simulink model "FusionMODEL_version1"  (R2018a)
settings: Solver=FixedStepAuto  StartTime=0.0  StopTime=SimulationTime  FixedStep=SamplingTime  RelTol=1e-3
undefined symbols (not defined in the file or in its folder): ACTIVATE_CAM, ACTIVATE_RAD, CAM1_detTimeStamp, CAM1_MeasNoise, CAM1_objClassID, CAM1_PX, CAM1_PY, CAM1_VX, CAM1_VY, CAM2_detTimeStamp, CAM2_MeasNoise, CAM2_objClassID, CAM2_PX, CAM2_PY, CAM2_VX, CAM2_VY, CAM3_detTimeStamp, CAM3_MeasNoise, CAM3_objClassID, CAM3_PX, CAM3_PY, CAM3_VX, CAM3_VY, CAM4_detTimeStamp, CAM4_MeasNoise, CAM4_objClassID, CAM4_PX, CAM4_PY, CAM4_VX, CAM4_VY, CAM5_detTimeStamp, CAM5_MeasNoise, CAM5_objClassID, CAM5_PX, CAM5_PY, CAM5_VX, CAM5_VY, CAM6_detTimeStamp, CAM6_MeasNoise, CAM6_objClassID, CAM6_PX, CAM6_PY, CAM6_VX, CAM6_VY, CAM7_detTimeStamp, CAM7_MeasNoise, CAM7_objClassID, CAM7_PX, CAM7_PY, CAM7_VX, CAM7_VY, CAM8_detTimeStamp, CAM8_MeasNoise, CAM8_objClassID, CAM8_PX, CAM8_PY, CAM8_VX, CAM8_VY, CAM_nMeas, CAM_TYPE ... (+151)
libraries: simulink_extras x2
(part 6 of 6)

== system FusionMODEL_version1/SENSOR_MEASUREMENTS/RADAR_CAMERA_EGO_SENSOR_INTERFACE/RoadSensors/Camera6/ExtractMeasParam1 ==
  idx : Inport
  time : Inport  Port=2
  Constant : Constant  Value=LINE_CURVATURE_CAM6
  Constant1 : Constant  Value=LINE_CURVDERIVATIVE_CAM6
  Constant2 : Constant  Value=LINE_CURVELENGTH_CAM6
  Constant3 : Constant  Value=LINE_HEADINGANGLE_CAM6
  Constant4 : Constant  Value=LINE_LATERALOFFSET_CAM6
  Constant5 : Constant  Value=LINE_XMIN_CAM6
  Constant6 : Constant  Value=LINE_detTimeStamp_CAM6
  Constant7 : Constant  Value=LINE_XMAX_CAM6
  Constant8 : Constant  Value=LINE_WIDTH_CAM6
  CurvLength : Selector  NumberOfDimensions=2  InputPortWidth=3  IndexOptions=Index vector (port),Index vector (port)  Indices=[1 3],1  OutputSizes=1,1
  Curvature : Selector  NumberOfDimensions=2  InputPortWidth=3  IndexOptions=Index vector (port),Index vector (port)  Indices=[1 3],1  OutputSizes=1,1
  CurvatureRate : Selector  NumberOfDimensions=2  InputPortWidth=3  IndexOptions=Index vector (port),Index vector (port)  Indices=[1 3],1  OutputSizes=1,1
  HeadingAngle : Selector  NumberOfDimensions=2  InputPortWidth=3  IndexOptions=Index vector (port),Index vector (port)  Indices=[1 3],1  OutputSizes=1,1
  LateralOffset : Selector  NumberOfDimensions=2  InputPortWidth=3  IndexOptions=Index vector (port),Index vector (port)  Indices=[1 3],1  OutputSizes=1,1
  lineWidth : Selector  NumberOfDimensions=2  InputPortWidth=3  IndexOptions=Index vector (port),Index vector (port)  Indices=[1 3],1  OutputSizes=1,1
  minValidX : Selector  NumberOfDimensions=2  InputPortWidth=3  IndexOptions=Index vector (port),Index vector (port)  Indices=[1 3],1  OutputSizes=1,1
  minValidY : Selector  NumberOfDimensions=2  InputPortWidth=3  IndexOptions=Index vector (port),Index vector (port)  Indices=[1 3],1  OutputSizes=1,1
  timeStamp : Selector  NumberOfDimensions=2  InputPortWidth=3  IndexOptions=Select all,Index vector (port)  Indices=[1 3],1  OutputSizes=1,1
  curvature : Outport
  curvRate : Outport  Port=2
  curvLength : Outport  Port=3
  headingAngle : Outport  Port=4
  lateralOffset : Outport  Port=5
  xmin : Outport  Port=6
  xmax : Outport  Port=7
  lineMarkWidth : Outport  Port=8
  measCaptureTime : Outport  Port=9
  wires:
  Constant3/1 -> HeadingAngle/1
  Constant2/1 -> CurvLength/1
  HeadingAngle/1 -> headingAngle/1
  Constant/1 -> Curvature/1
  Constant1/1 -> CurvatureRate/1
  CurvLength/1 -> curvLength/1
  Curvature/1 -> curvature/1
  CurvatureRate/1 -> curvRate/1
  Constant4/1 -> LateralOffset/1
  Constant5/1 -> minValidX/1
  Constant6/1 -> timeStamp/1
  timeStamp/1 -> measCaptureTime/1
  minValidX/1 -> xmin/1
  LateralOffset/1 -> lateralOffset/1
  minValidY/1 -> xmax/1
  Constant7/1 -> minValidY/1
  lineWidth/1 -> lineMarkWidth/1
  time/1 -> minValidX/2, minValidY/2, lineWidth/2, timeStamp/2, LateralOffset/2, HeadingAngle/2, CurvLength/2, CurvatureRate/2, Curvature/2
  idx/1 -> minValidX/3, lineWidth/3, minValidY/3, LateralOffset/3, HeadingAngle/3, CurvLength/3, CurvatureRate/3, Curvature/3
  Constant8/1 -> lineWidth/1

== system FusionMODEL_version1/SENSOR_MEASUREMENTS/RADAR_CAMERA_EGO_SENSOR_INTERFACE/RoadSensors/Camera6/IsValid2 ==
  LineID : Inport
  curvature : Inport  Port=2
  curvatureRate : Inport  Port=3
  curvLength : Inport  Port=4
  HeadingAngle : Inport  Port=5
  Abs{,1..3} (4 alike) : Abs
  Add : Sum  Inputs=++++
  Constant : Constant  Value=uint16(0)
  Data Type Conversion : DataTypeConversion  OutDataTypeStr=uint16
  Switch : Switch  Threshold=0.000001
  validID : Outport
  wires:
  Add/1 -> Switch/2
  Abs2/1 -> Add/3
  Constant/1 -> Switch/3
  Abs/1 -> Add/1
  curvature/1 -> Abs/1
  Abs3/1 -> Add/4
  Abs1/1 -> Add/2
  HeadingAngle/1 -> Abs3/1
  curvatureRate/1 -> Abs1/1
  curvLength/1 -> Abs2/1
  LineID/1 -> Data Type Conversion/1
  Switch/1 -> validID/1
  Data Type Conversion/1 -> Switch/1

== system FusionMODEL_version1/SENSOR_MEASUREMENTS/RADAR_CAMERA_EGO_SENSOR_INTERFACE/RoadSensors/Camera6/Subsystem1 ==
  CameraLineCoeff : Inport
  curv : Inport  Port=2
  curvRate : Inport  Port=3
  curvLen : Inport  Port=4
  alpha : Inport  Port=5
  ValidID : Inport  Port=6
  lateralOffset : Inport  Port=7
  xmin : Inport  Port=8
  xmax : Inport  Port=9
  lineWidth : Inport  Port=10
  TIME_STAMP : Inport  Port=11
  iter : Inport  Port=12
  Assignment : Assignment  DiagnosticForDimensions=Warning  IndexOptions=Index vector (port)  Indices=1  OutputSizes=1
  Bus Creator1 : BusCreator  Inputs=11  OutDataTypeStr=Bus: LineMeasParam  NonVirtualBus=on
  Bus Creator2 : BusCreator  Inputs=11  OutDataTypeStr=Bus: LineMeasParam  NonVirtualBus=on
  Constant1 : Constant  Value=single(10)
  Constant14 : Constant  Value=uint8(6)
  Constant2 : Constant  Value=single(10)
  Constant{35..39,43} (6 alike) : Constant  Value=single(0)
  Constant44 : Constant  Value=single(10)
  Switch : Switch  Criteria=u2 ~= 0
  C1 : Outport
  wires:
  Bus Creator1/1 -> Switch/3
  ValidID/1 -> Bus Creator1/2, Switch/2, Bus Creator2/2  "lineID"
  Bus Creator2/1 -> Switch/1
  CameraLineCoeff/1 -> Assignment/1
  Switch/1 -> Assignment/2
  iter/1 -> Assignment/3
  Assignment/1 -> C1/1
  TIME_STAMP/1 -> Bus Creator2/1  "TimeStamp"
  curv/1 -> Bus Creator2/4  "curvature"
  curvRate/1 -> Bus Creator2/5  "curvatureRate"
  curvLen/1 -> Bus Creator2/6  "curveLength"
  alpha/1 -> Bus Creator2/7  "HeadingAngle"
  lateralOffset/1 -> Bus Creator2/8  "LateralOffset"
  lineWidth/1 -> Bus Creator2/11  "LineMarkWidth"
  xmax/1 -> Bus Creator2/10  "validMinLongCoordLine"
  xmin/1 -> Bus Creator2/9  "validMaxLongCoordLine"
  Constant35/1 -> Bus Creator1/1  "TimeStamp"
  Constant14/1 -> Bus Creator2/3, Bus Creator1/3  "cameraID"
  Constant36/1 -> Bus Creator1/4  "curvature"
  Constant37/1 -> Bus Creator1/5  "curvatureRate"
  Constant38/1 -> Bus Creator1/6  "curveLength"
  Constant39/1 -> Bus Creator1/7  "HeadingAngle"
  Constant43/1 -> Bus Creator1/8  "LateralOffset"
  Constant44/1 -> Bus Creator1/9  "validMaxLongCoordLine"
  Constant1/1 -> Bus Creator1/10  "validMinLongCoordLine"
  Constant2/1 -> Bus Creator1/11  "LineMarkWidth"

== system FusionMODEL_version1/SENSOR_MEASUREMENTS/RADAR_CAMERA_EGO_SENSOR_INTERFACE/RoadSensors/Camera7/ExtractMeasParam1 ==
  idx : Inport
  time : Inport  Port=2
  Constant : Constant  Value=LINE_CURVATURE_CAM7
  Constant1 : Constant  Value=LINE_CURVDERIVATIVE_CAM7
  Constant2 : Constant  Value=LINE_CURVELENGTH_CAM7
  Constant3 : Constant  Value=LINE_HEADINGANGLE_CAM7
  Constant4 : Constant  Value=LINE_LATERALOFFSET_CAM7
  Constant5 : Constant  Value=LINE_XMIN_CAM7
  Constant6 : Constant  Value=LINE_detTimeStamp_CAM7
  Constant7 : Constant  Value=LINE_XMAX_CAM7
  Constant8 : Constant  Value=LINE_WIDTH_CAM7
  CurvLength : Selector  NumberOfDimensions=2  InputPortWidth=3  IndexOptions=Index vector (port),Index vector (port)  Indices=[1 3],1  OutputSizes=1,1
  Curvature : Selector  NumberOfDimensions=2  InputPortWidth=3  IndexOptions=Index vector (port),Index vector (port)  Indices=[1 3],1  OutputSizes=1,1
  CurvatureRate : Selector  NumberOfDimensions=2  InputPortWidth=3  IndexOptions=Index vector (port),Index vector (port)  Indices=[1 3],1  OutputSizes=1,1
  HeadingAngle : Selector  NumberOfDimensions=2  InputPortWidth=3  IndexOptions=Index vector (port),Index vector (port)  Indices=[1 3],1  OutputSizes=1,1
  LateralOffset : Selector  NumberOfDimensions=2  InputPortWidth=3  IndexOptions=Index vector (port),Index vector (port)  Indices=[1 3],1  OutputSizes=1,1
  lineWidth : Selector  NumberOfDimensions=2  InputPortWidth=3  IndexOptions=Index vector (port),Index vector (port)  Indices=[1 3],1  OutputSizes=1,1
  minValidX : Selector  NumberOfDimensions=2  InputPortWidth=3  IndexOptions=Index vector (port),Index vector (port)  Indices=[1 3],1  OutputSizes=1,1
  minValidY : Selector  NumberOfDimensions=2  InputPortWidth=3  IndexOptions=Index vector (port),Index vector (port)  Indices=[1 3],1  OutputSizes=1,1
  timeStamp : Selector  NumberOfDimensions=2  InputPortWidth=3  IndexOptions=Select all,Index vector (port)  Indices=[1 3],1  OutputSizes=1,1
  curvature : Outport
  curvRate : Outport  Port=2
  curvLength : Outport  Port=3
  headingAngle : Outport  Port=4
  lateralOffset : Outport  Port=5
  xmin : Outport  Port=6
  xmax : Outport  Port=7
  lineMarkWidth : Outport  Port=8
  measCaptureTime : Outport  Port=9
  wires:
  Constant3/1 -> HeadingAngle/1
  Constant2/1 -> CurvLength/1
  HeadingAngle/1 -> headingAngle/1
  Constant/1 -> Curvature/1
  Constant1/1 -> CurvatureRate/1
  CurvLength/1 -> curvLength/1
  Curvature/1 -> curvature/1
  CurvatureRate/1 -> curvRate/1
  Constant4/1 -> LateralOffset/1
  Constant5/1 -> minValidX/1
  Constant6/1 -> timeStamp/1
  timeStamp/1 -> measCaptureTime/1
  minValidX/1 -> xmin/1
  LateralOffset/1 -> lateralOffset/1
  minValidY/1 -> xmax/1
  Constant7/1 -> minValidY/1
  lineWidth/1 -> lineMarkWidth/1
  time/1 -> minValidX/2, minValidY/2, lineWidth/2, timeStamp/2, LateralOffset/2, HeadingAngle/2, CurvLength/2, CurvatureRate/2, Curvature/2
  idx/1 -> minValidX/3, lineWidth/3, minValidY/3, LateralOffset/3, HeadingAngle/3, CurvLength/3, CurvatureRate/3, Curvature/3
  Constant8/1 -> lineWidth/1

== system FusionMODEL_version1/SENSOR_MEASUREMENTS/RADAR_CAMERA_EGO_SENSOR_INTERFACE/RoadSensors/Camera7/IsValid2 ==
  LineID : Inport
  curvature : Inport  Port=2
  curvatureRate : Inport  Port=3
  curvLength : Inport  Port=4
  HeadingAngle : Inport  Port=5
  Abs{,1..3} (4 alike) : Abs
  Add : Sum  Inputs=++++
  Constant : Constant  Value=uint16(0)
  Data Type Conversion : DataTypeConversion  OutDataTypeStr=uint16
  Switch : Switch  Threshold=0.000001
  validID : Outport
  wires:
  Add/1 -> Switch/2
  Abs2/1 -> Add/3
  Constant/1 -> Switch/3
  Abs/1 -> Add/1
  curvature/1 -> Abs/1
  Abs3/1 -> Add/4
  Abs1/1 -> Add/2
  HeadingAngle/1 -> Abs3/1
  curvatureRate/1 -> Abs1/1
  curvLength/1 -> Abs2/1
  LineID/1 -> Data Type Conversion/1
  Switch/1 -> validID/1
  Data Type Conversion/1 -> Switch/1

== system FusionMODEL_version1/SENSOR_MEASUREMENTS/RADAR_CAMERA_EGO_SENSOR_INTERFACE/RoadSensors/Camera7/Subsystem1 ==
  CameraLineCoeff : Inport
  curv : Inport  Port=2
  curvRate : Inport  Port=3
  curvLen : Inport  Port=4
  alpha : Inport  Port=5
  ValidID : Inport  Port=6
  lateralOffset : Inport  Port=7
  xmin : Inport  Port=8
  xmax : Inport  Port=9
  lineWidth : Inport  Port=10
  TIME_STAMP : Inport  Port=11
  iter : Inport  Port=12
  Assignment : Assignment  DiagnosticForDimensions=Warning  IndexOptions=Index vector (port)  Indices=1  OutputSizes=1
  Bus Creator1 : BusCreator  Inputs=11  OutDataTypeStr=Bus: LineMeasParam  NonVirtualBus=on
  Bus Creator2 : BusCreator  Inputs=11  OutDataTypeStr=Bus: LineMeasParam  NonVirtualBus=on
  Constant1 : Constant  Value=single(10)
  Constant14 : Constant  Value=uint8(7)
  Constant2 : Constant  Value=single(10)
  Constant{35..39,43} (6 alike) : Constant  Value=single(0)
  Constant44 : Constant  Value=single(10)
  Switch : Switch  Criteria=u2 ~= 0
  C1 : Outport
  wires:
  Bus Creator1/1 -> Switch/3
  ValidID/1 -> Bus Creator1/2, Switch/2, Bus Creator2/2  "lineID"
  Bus Creator2/1 -> Switch/1
  CameraLineCoeff/1 -> Assignment/1
  Switch/1 -> Assignment/2
  iter/1 -> Assignment/3
  Assignment/1 -> C1/1
  TIME_STAMP/1 -> Bus Creator2/1  "TimeStamp"
  curv/1 -> Bus Creator2/4  "curvature"
  curvRate/1 -> Bus Creator2/5  "curvatureRate"
  curvLen/1 -> Bus Creator2/6  "curveLength"
  alpha/1 -> Bus Creator2/7  "HeadingAngle"
  lateralOffset/1 -> Bus Creator2/8  "LateralOffset"
  lineWidth/1 -> Bus Creator2/11  "LineMarkWidth"
  xmax/1 -> Bus Creator2/10  "validMinLongCoordLine"
  xmin/1 -> Bus Creator2/9  "validMaxLongCoordLine"
  Constant35/1 -> Bus Creator1/1  "TimeStamp"
  Constant14/1 -> Bus Creator2/3, Bus Creator1/3  "cameraID"
  Constant36/1 -> Bus Creator1/4  "curvature"
  Constant37/1 -> Bus Creator1/5  "curvatureRate"
  Constant38/1 -> Bus Creator1/6  "curveLength"
  Constant39/1 -> Bus Creator1/7  "HeadingAngle"
  Constant43/1 -> Bus Creator1/8  "LateralOffset"
  Constant44/1 -> Bus Creator1/9  "validMaxLongCoordLine"
  Constant1/1 -> Bus Creator1/10  "validMinLongCoordLine"
  Constant2/1 -> Bus Creator1/11  "LineMarkWidth"

== system FusionMODEL_version1/SENSOR_MEASUREMENTS/RADAR_CAMERA_EGO_SENSOR_INTERFACE/RoadSensors/Camera8/ExtractMeasParam1 ==
  idx : Inport
  time : Inport  Port=2
  Constant : Constant  Value=LINE_CURVATURE_CAM8
  Constant1 : Constant  Value=LINE_CURVDERIVATIVE_CAM8
  Constant2 : Constant  Value=LINE_CURVELENGTH_CAM8
  Constant3 : Constant  Value=LINE_HEADINGANGLE_CAM8
  Constant4 : Constant  Value=LINE_LATERALOFFSET_CAM8
  Constant5 : Constant  Value=LINE_XMIN_CAM8
  Constant6 : Constant  Value=LINE_detTimeStamp_CAM8
  Constant7 : Constant  Value=LINE_XMAX_CAM8
  Constant8 : Constant  Value=LINE_WIDTH_CAM8
  CurvLength : Selector  NumberOfDimensions=2  InputPortWidth=3  IndexOptions=Index vector (port),Index vector (port)  Indices=[1 3],1  OutputSizes=1,1
  Curvature : Selector  NumberOfDimensions=2  InputPortWidth=3  IndexOptions=Index vector (port),Index vector (port)  Indices=[1 3],1  OutputSizes=1,1
  CurvatureRate : Selector  NumberOfDimensions=2  InputPortWidth=3  IndexOptions=Index vector (port),Index vector (port)  Indices=[1 3],1  OutputSizes=1,1
  HeadingAngle : Selector  NumberOfDimensions=2  InputPortWidth=3  IndexOptions=Index vector (port),Index vector (port)  Indices=[1 3],1  OutputSizes=1,1
  LateralOffset : Selector  NumberOfDimensions=2  InputPortWidth=3  IndexOptions=Index vector (port),Index vector (port)  Indices=[1 3],1  OutputSizes=1,1
  lineWidth : Selector  NumberOfDimensions=2  InputPortWidth=3  IndexOptions=Index vector (port),Index vector (port)  Indices=[1 3],1  OutputSizes=1,1
  minValidX : Selector  NumberOfDimensions=2  InputPortWidth=3  IndexOptions=Index vector (port),Index vector (port)  Indices=[1 3],1  OutputSizes=1,1
  minValidY : Selector  NumberOfDimensions=2  InputPortWidth=3  IndexOptions=Index vector (port),Index vector (port)  Indices=[1 3],1  OutputSizes=1,1
  timeStamp : Selector  NumberOfDimensions=2  InputPortWidth=3  IndexOptions=Select all,Index vector (port)  Indices=[1 3],1  OutputSizes=1,1
  curvature : Outport
  curvRate : Outport  Port=2
  curvLength : Outport  Port=3
  headingAngle : Outport  Port=4
  lateralOffset : Outport  Port=5
  xmin : Outport  Port=6
  xmax : Outport  Port=7
  lineMarkWidth : Outport  Port=8
  measCaptureTime : Outport  Port=9
  wires:
  Constant3/1 -> HeadingAngle/1
  Constant2/1 -> CurvLength/1
  HeadingAngle/1 -> headingAngle/1
  Constant/1 -> Curvature/1
  Constant1/1 -> CurvatureRate/1
  CurvLength/1 -> curvLength/1
  Curvature/1 -> curvature/1
  CurvatureRate/1 -> curvRate/1
  Constant4/1 -> LateralOffset/1
  Constant5/1 -> minValidX/1
  Constant6/1 -> timeStamp/1
  timeStamp/1 -> measCaptureTime/1
  minValidX/1 -> xmin/1
  LateralOffset/1 -> lateralOffset/1
  minValidY/1 -> xmax/1
  Constant7/1 -> minValidY/1
  lineWidth/1 -> lineMarkWidth/1
  time/1 -> minValidX/2, minValidY/2, lineWidth/2, timeStamp/2, LateralOffset/2, HeadingAngle/2, CurvLength/2, CurvatureRate/2, Curvature/2
  idx/1 -> minValidX/3, lineWidth/3, minValidY/3, LateralOffset/3, HeadingAngle/3, CurvLength/3, CurvatureRate/3, Curvature/3
  Constant8/1 -> lineWidth/1

== system FusionMODEL_version1/SENSOR_MEASUREMENTS/RADAR_CAMERA_EGO_SENSOR_INTERFACE/RoadSensors/Camera8/IsValid2 ==
  LineID : Inport
  curvature : Inport  Port=2
  curvatureRate : Inport  Port=3
  curvLength : Inport  Port=4
  HeadingAngle : Inport  Port=5
  Abs{,1..3} (4 alike) : Abs
  Add : Sum  Inputs=++++
  Constant : Constant  Value=uint16(0)
  Data Type Conversion : DataTypeConversion  OutDataTypeStr=uint16
  Switch : Switch  Threshold=0.000001
  validID : Outport
  wires:
  Add/1 -> Switch/2
  Abs2/1 -> Add/3
  Constant/1 -> Switch/3
  Abs/1 -> Add/1
  curvature/1 -> Abs/1
  Abs3/1 -> Add/4
  Abs1/1 -> Add/2
  HeadingAngle/1 -> Abs3/1
  curvatureRate/1 -> Abs1/1
  curvLength/1 -> Abs2/1
  LineID/1 -> Data Type Conversion/1
  Switch/1 -> validID/1
  Data Type Conversion/1 -> Switch/1

== system FusionMODEL_version1/SENSOR_MEASUREMENTS/RADAR_CAMERA_EGO_SENSOR_INTERFACE/RoadSensors/Camera8/Subsystem1 ==
  CameraLineCoeff : Inport
  curv : Inport  Port=2
  curvRate : Inport  Port=3
  curvLen : Inport  Port=4
  alpha : Inport  Port=5
  ValidID : Inport  Port=6
  lateralOffset : Inport  Port=7
  xmin : Inport  Port=8
  xmax : Inport  Port=9
  lineWidth : Inport  Port=10
  TIME_STAMP : Inport  Port=11
  iter : Inport  Port=12
  Assignment : Assignment  DiagnosticForDimensions=Warning  IndexOptions=Index vector (port)  Indices=1  OutputSizes=1
  Bus Creator1 : BusCreator  Inputs=11  OutDataTypeStr=Bus: LineMeasParam  NonVirtualBus=on
  Bus Creator2 : BusCreator  Inputs=11  OutDataTypeStr=Bus: LineMeasParam  NonVirtualBus=on
  Constant1 : Constant  Value=single(10)
  Constant14 : Constant  Value=uint8(8)
  Constant2 : Constant  Value=single(10)
  Constant{35..39,43} (6 alike) : Constant  Value=single(0)
  Constant44 : Constant  Value=single(10)
  Switch : Switch  Criteria=u2 ~= 0
  C1 : Outport
  wires:
  Bus Creator1/1 -> Switch/3
  ValidID/1 -> Bus Creator1/2, Switch/2, Bus Creator2/2  "lineID"
  Bus Creator2/1 -> Switch/1
  CameraLineCoeff/1 -> Assignment/1
  Switch/1 -> Assignment/2
  iter/1 -> Assignment/3
  Assignment/1 -> C1/1
  TIME_STAMP/1 -> Bus Creator2/1  "TimeStamp"
  curv/1 -> Bus Creator2/4  "curvature"
  curvRate/1 -> Bus Creator2/5  "curvatureRate"
  curvLen/1 -> Bus Creator2/6  "curveLength"
  alpha/1 -> Bus Creator2/7  "HeadingAngle"
  lateralOffset/1 -> Bus Creator2/8  "LateralOffset"
  lineWidth/1 -> Bus Creator2/11  "LineMarkWidth"
  xmax/1 -> Bus Creator2/10  "validMinLongCoordLine"
  xmin/1 -> Bus Creator2/9  "validMaxLongCoordLine"
  Constant35/1 -> Bus Creator1/1  "TimeStamp"
  Constant14/1 -> Bus Creator2/3, Bus Creator1/3  "cameraID"
  Constant36/1 -> Bus Creator1/4  "curvature"
  Constant37/1 -> Bus Creator1/5  "curvatureRate"
  Constant38/1 -> Bus Creator1/6  "curveLength"
  Constant39/1 -> Bus Creator1/7  "HeadingAngle"
  Constant43/1 -> Bus Creator1/8  "LateralOffset"
  Constant44/1 -> Bus Creator1/9  "validMaxLongCoordLine"
  Constant1/1 -> Bus Creator1/10  "validMinLongCoordLine"
  Constant2/1 -> Bus Creator1/11  "LineMarkWidth"

== system FusionMODEL_version1/OBJECT_TRACKER_SENSOR_FUSION/SET_SENSOR_CALLIBRATION_PARAMETER/SET_CAMERA_SENSOR_PARAM/SET_CAMERA_EXTRINSIC_PARAM/SET_CAMERA_EXTRINSIC_PARAM/CreateRotationMatTranslationVector ==
  yawInstall : Inport
  xMount : Inport  Port=2
  yMount : Inport  Port=3
  Cos : Trigonometry  Operator=cos
  Cos2 : Trigonometry
  Degrees to Radians : simulink_extras/Transformations/Degrees to Radians
  Gain1 : Gain  Gain=-1
  Gain2 : Gain  Gain=ROT_CONVENTION
  Mux : Mux
  Mux1 : Mux  Inputs=2
  Reshape : Reshape  OutputDimensionality=Customize  OutputDimensions=[2 2]
  Reshape1 : Reshape  OutputDimensionality=Column vector (2-D)  OutputDimensions=[2 2]
  RotMatrx : Outport
  TranslationVector : Outport  Port=2
  wires:
  Cos/1 -> [cos_theta], Mux/1
  [cos_theta] -> Mux/4
  Reshape/1 -> RotMatrx/1
  Degrees to Radians/1 -> Cos2/1, Cos/1
  Mux/1 -> Reshape/1
  Cos2/1 -> Mux/2, Gain1/1
  xMount/1 -> Mux1/1
  yMount/1 -> Mux1/2
  Mux1/1 -> Reshape1/1
  Reshape1/1 -> TranslationVector/1
  Gain1/1 -> Mux/3
  yawInstall/1 -> Gain2/1
  Gain2/1 -> Degrees to Radians/1

== system FusionMODEL_version1/OBJECT_TRACKER_SENSOR_FUSION/SET_SENSOR_CALLIBRATION_PARAMETER/SET_RADAR_SENSOR_PARAM/SET_RADAR_EXTRINSIC_PARAM/SET_RADAR_EXTRINSIC_PARAM/CREATE_ROTATION_MATRIX_TRANSLATION_VECTOR ==
  yawInstall : Inport
  xMount : Inport  Port=2
  yMount : Inport  Port=3
  Cos : Trigonometry  Operator=cos
  Cos2 : Trigonometry
  Degrees to Radians : simulink_extras/Transformations/Degrees to Radians
  Gain1 : Gain  Gain=-1
  Gain2 : Gain  Gain=ROT_CONVENTION
  Mux : Mux
  Mux1 : Mux  Inputs=2
  Reshape : Reshape  OutputDimensionality=Customize  OutputDimensions=[2 2]
  Reshape1 : Reshape  OutputDimensionality=Column vector (2-D)  OutputDimensions=[2 2]
  RotMatrx : Outport
  TranslationVector : Outport  Port=2
  wires:
  Cos/1 -> [cos_theta], Mux/1
  [cos_theta] -> Mux/4
  Reshape/1 -> RotMatrx/1
  Degrees to Radians/1 -> Cos2/1, Cos/1
  Mux/1 -> Reshape/1
  Cos2/1 -> Mux/2, Gain1/1
  xMount/1 -> Mux1/1
  yMount/1 -> Mux1/2
  Mux1/1 -> Reshape1/1
  Reshape1/1 -> TranslationVector/1
  Gain1/1 -> Mux/3
  yawInstall/1 -> Gain2/1
  Gain2/1 -> Degrees to Radians/1

== system FusionMODEL_version1/OBJECT_TRACKER_SENSOR_FUSION/SPATIAL_ALLIGNMENT/CAMERA_MEASUREMENTS_SPATIAL_ALLIGNMENT/For Iterator Subsystem/For Iterator Subsystem/CoordinateTransformation1 ==
  meas : Inport
  SensorParam : Inport  Port=2
  Action Port : ActionPort  ActionType=then
  InfoExtractor : Subsystem
  Meas_Noise_Cov_Transformation : Subsystem
  Position_Transformation : Subsystem
  Subsystem : Subsystem
  Velocity_Transformation : Subsystem
  measUpd : Outport
  wires:
  meas/1 -> InfoExtractor/1(In1)
  SensorParam/1 -> InfoExtractor/2(In2)
  Velocity_Transformation/1(VelXcts) -> [VxCTS]  "vxCTS"
  InfoExtractor/5(RotMat2D) -> Velocity_Transformation/3(RotMatrix2D), Meas_Noise_Cov_Transformation/1(RotMatrix), [RotMat]
  InfoExtractor/4(<vy>) -> Velocity_Transformation/2(Vy)
  InfoExtractor/3(<vx>) -> Velocity_Transformation/1(Vx)
  InfoExtractor/1(<px>) -> Position_Transformation/1(Px)
  InfoExtractor/2(<py>) -> Position_Transformation/2(Py)
  InfoExtractor/7(MeasNoiseCov) -> Meas_Noise_Cov_Transformation/2(MeasCovarience)
  [RotMat] -> Position_Transformation/3(RotationMat)
  [TransVector] -> Position_Transformation/4(TranslationVector)
  InfoExtractor/6(TransVec2D) -> [TransVector]
  Position_Transformation/1(PosXcts) -> Subsystem/1(pxCTS)
  Meas_Noise_Cov_Transformation/1(MeasCovTransformed) -> Subsystem/5(covCTS)
  Position_Transformation/2(PosYcts) -> Subsystem/2(pyCTS)
  Velocity_Transformation/2(VelYcts) -> [VyCTS]  "vyCTS"
  [VxCTS] -> Subsystem/3(vxCTS)
  [VyCTS] -> Subsystem/4(vyCTS)
  Subsystem/1(measUpd) -> measUpd/1

== system FusionMODEL_version1/OBJECT_TRACKER_SENSOR_FUSION/SPATIAL_ALLIGNMENT/CAMERA_MEASUREMENTS_SPATIAL_ALLIGNMENT/For Iterator Subsystem/For Iterator Subsystem/SetMeasurement ==
  measTransformed : Inport
  measID : Inport  Port=2
  CamCANidx : Inport  Port=3
  CameraMeasCAN : Inport  Port=4
  CameraMeasCTSMat : Inport  Port=5
  Assignment1 : Assignment  NumberOfDimensions=2  DiagnosticForDimensions=Warning  IndexOptions=Index vector (dialog),Index vector (port)  Indices=1:8,1  OutputSizes=1,1
  Bus Selector : BusSelector  OutputSignals=measID,cameraID
  Bus to Vector : BusToVector
  Constant : Constant  Value=single(zeros(8,1))
  Data Type Conversion : DataTypeConversion  OutDataTypeStr=single
  Data Type Conversion1 : DataTypeConversion  OutDataTypeStr=single
  Mux : Mux  Inputs=3
  Reshape : Reshape  OutputDimensionality=Column vector (2-D)
  Switch : Switch  Criteria=u2 ~= 0
  Unit Delay : UnitDelay  InitialCondition=single(zeros(8, 200))  SampleTime=-1
  CameraCTSMatUpd : Outport
  wires:
  CameraMeasCTSMat/1 -> Unit Delay/1
  measID/1 -> Switch/2
  Constant/1 -> Switch/3
  Switch/1 -> Assignment1/2
  CamCANidx/1 -> Assignment1/3
  CameraMeasCAN/1 -> Bus Selector/1
  Unit Delay/1 -> Assignment1/1
  measTransformed/1 -> Bus to Vector/1
  Assignment1/1 -> CameraCTSMatUpd/1
  Bus Selector/1 -> Data Type Conversion/1  "<measID>"
  Bus Selector/2 -> Data Type Conversion1/1  "<cameraID>"
  Data Type Conversion1/1 -> Mux/3
  Data Type Conversion/1 -> Mux/2
  Bus to Vector/1 -> Mux/1
  Mux/1 -> Reshape/1
  Reshape/1 -> Switch/1

== system FusionMODEL_version1/OBJECT_TRACKER_SENSOR_FUSION/SPATIAL_ALLIGNMENT/CAMERA_MEASUREMENTS_SPATIAL_ALLIGNMENT/For Iterator Subsystem/For Iterator Subsystem/SetMeasurement1 ==
  measTransformed : Inport
  measID : Inport  Port=2
  CamCANidx : Inport  Port=3
  CameraMeasCAN : Inport  Port=4
  CameraMeasCTSMat : Inport  Port=5
  CameraMeasCTSNoiseMat : Inport  Port=6
  CameraMeasCTSRef : Inport  Port=7
  Assignment1 : Assignment  NumberOfDimensions=2  DiagnosticForDimensions=Warning  IndexOptions=Assign all,Index vector (port)  Indices=1:2,1  OutputSizes=1,1
  Assignment2 : Assignment  NumberOfDimensions=3  DiagnosticForDimensions=Warning  IndexOptions=Assign all,Assign all,Index vector (port)  Indices=1:8,1,1  OutputSizes=1,1,1
  Assignment3 : Assignment  NumberOfDimensions=2  DiagnosticForDimensions=Warning  IndexOptions=Assign all,Index vector (port)  Indices=1:8,1  OutputSizes=1,1
  Bus Selector : BusSelector  OutputSignals=measID,cameraID
  Bus Selector1 : BusSelector  OutputSignals=stateCTS,covCTS
  Constant : Constant  Value=single(zeros(2,1))
  Constant1 : Constant  Value=single(zeros(2,2))
  Constant2 : Constant  Value=uint16(zeros(2,1))
  Data Type Conversion : DataTypeConversion  OutDataTypeStr=uint16
  Mux : Mux  Inputs=2
  Reshape : Reshape  OutputDimensionality=Column vector (2-D)
  Switch : Switch  Criteria=u2 ~= 0
  Switch1 : Switch  Criteria=u2 ~= 0
  Switch2 : Switch  Criteria=u2 ~= 0
  Unit Delay : UnitDelay  InitialCondition=single(zeros(2, 200))  SampleTime=-1
  Unit Delay1 : UnitDelay  InitialCondition=single(zeros(2, 2, 200))  SampleTime=-1
  Unit Delay2 : UnitDelay  InitialCondition=uint16(zeros(2, 200))  SampleTime=-1
  CameraCTSMatUpd : Outport
  CameraCTSNoiseCovMatUpd : Outport  Port=2
  CameraCTSRefUpd : Outport  Port=3
  wires:
  CameraMeasCTSMat/1 -> Unit Delay/1
  measID/1 -> Switch/2, Switch2/2, Switch1/2
  Constant/1 -> Switch/3
  Switch/1 -> Assignment1/2
  CamCANidx/1 -> [idx], Assignment1/3
  CameraMeasCAN/1 -> Bus Selector/1
  Unit Delay/1 -> Assignment1/1
  Assignment1/1 -> CameraCTSMatUpd/1
  Bus Selector/1 -> Mux/1  "<measID>"
  Bus Selector/2 -> Data Type Conversion/1  "<cameraID>"
  Mux/1 -> Reshape/1
  CameraMeasCTSNoiseMat/1 -> Unit Delay1/1
  Unit Delay1/1 -> Assignment2/1
  Switch1/1 -> Assignment2/2
  measTransformed/1 -> Bus Selector1/1
  Bus Selector1/1 -> Switch/1  "<stateCTS>"
  Constant1/1 -> Switch1/3
  Bus Selector1/2 -> [CTSNoiseCov]  "<covCTS>"
  [CTSNoiseCov] -> Switch1/1
  [idx] -> Assignment2/3
  Switch2/1 -> Assignment3/2
  Constant2/1 -> Switch2/3
  [idx] -> Assignment3/3
  Unit Delay2/1 -> Assignment3/1
  CameraMeasCTSRef/1 -> Unit Delay2/1
  Reshape/1 -> [CTSRef]
  [CTSRef] -> Switch2/1
  Assignment2/1 -> CameraCTSNoiseCovMatUpd/1
  Assignment3/1 -> CameraCTSRefUpd/1
  Data Type Conversion/1 -> Mux/2

== system FusionMODEL_version1/OBJECT_TRACKER_SENSOR_FUSION/SPATIAL_ALLIGNMENT/CAMERA_MEASUREMENTS_SPATIAL_ALLIGNMENT/For Iterator Subsystem/For Iterator Subsystem/Subsystem ==
  measCAN : Inport
  measIdx : Inport  Port=2
  Add : Sum
  Bus Selector : BusSelector  OutputSignals=measID
  Constant : Constant  Value=int32(0)
  Constant2 : Constant  Value=int32(1)
  If : If  IfExpression=u1 ~= 0  ShowElse=off
  Selector : Selector  NumberOfDimensions=2  InputPortWidth=3  IndexOptions=Select all,Index vector (port)  Indices=[1 3],1  OutputSizes=1,1
  Switch : Switch  Criteria=u2 ~= 0
  Unit Delay : UnitDelay  InitialCondition=int32(0)  SampleTime=-1
  isValid : Outport
  measID : Outport  Port=2
  nValidMeasCnt : Outport  Port=3
  meas_i : Outport  Port=4
  wires:
  measIdx/1 -> Selector/2
  Selector/1 -> meas_i/1, Bus Selector/1
  measCAN/1 -> Selector/1
  If/1 -> isValid/1
  Switch/1 -> Add/1
  Bus Selector/1 -> measID/1, If/1, Switch/2  "<measID>"
  Constant2/1 -> Switch/1
  Unit Delay/1 -> Add/2
  Constant/1 -> Switch/3
  Add/1 -> nValidMeasCnt/1, Unit Delay/1

== system FusionMODEL_version1/OBJECT_TRACKER_SENSOR_FUSION/SPATIAL_ALLIGNMENT/RADAR_MEASUREMENTS_SPATIAL_ALLIGNMENT/RADAR_MEASUREMENTS_SPATIAL_ALLIGNMENT/COORDINATE_TRANSFORMATION/COORDINATE_TRANSFORMATION ==
  meas : Inport
  SensorParam : Inport  Port=2
  Action Port : ActionPort  ActionType=then
  GET_DATA : Subsystem
  MEAS_NOISE_COV_TRANSFORMATION : Subsystem
  POSITION_TRANSFORMATION : Subsystem
  SET_DATA : Subsystem
  VELOCITY_TRANSFORMATION : Subsystem
  measUpd : Outport
  wires:
  meas/1 -> GET_DATA/1(In1)
  SensorParam/1 -> GET_DATA/2(In2)
  VELOCITY_TRANSFORMATION/1(VelXcts) -> [VxCTS]  "vxCTS"
  GET_DATA/5(RotMat2D) -> VELOCITY_TRANSFORMATION/3(RotMatrix2D), MEAS_NOISE_COV_TRANSFORMATION/1(RotMatrix), [RotMat]
  GET_DATA/4(<vy>) -> VELOCITY_TRANSFORMATION/2(Vy)
  GET_DATA/3(<vx>) -> VELOCITY_TRANSFORMATION/1(Vx)
  GET_DATA/1(<px>) -> POSITION_TRANSFORMATION/1(Px)
  GET_DATA/2(<py>) -> POSITION_TRANSFORMATION/2(Py)
  GET_DATA/7(MeasNoiseCov) -> MEAS_NOISE_COV_TRANSFORMATION/2(MeasCovarience)
  [RotMat] -> POSITION_TRANSFORMATION/3(RotationMat)
  [TransVector] -> POSITION_TRANSFORMATION/4(TranslationVector)
  GET_DATA/6(TransVec2D) -> [TransVector]
  POSITION_TRANSFORMATION/1(PosXcts) -> SET_DATA/1(pxCTS)
  MEAS_NOISE_COV_TRANSFORMATION/1(MeasCovTransformed) -> SET_DATA/5(covCTS)
  POSITION_TRANSFORMATION/2(PosYcts) -> SET_DATA/2(pyCTS)
  VELOCITY_TRANSFORMATION/2(VelYcts) -> [VyCTS]  "vyCTS"
  [VxCTS] -> SET_DATA/3(vxCTS)
  [VyCTS] -> SET_DATA/4(vyCTS)
  SET_DATA/1(measUpd) -> measUpd/1

== system FusionMODEL_version1/OBJECT_TRACKER_SENSOR_FUSION/SPATIAL_ALLIGNMENT/RADAR_MEASUREMENTS_SPATIAL_ALLIGNMENT/RADAR_MEASUREMENTS_SPATIAL_ALLIGNMENT/COORDINATE_TRANSFORMATION/GET_DATA ==
  measCAN : Inport
  measIdx : Inport  Port=2
  Add : Sum
  Bus Selector : BusSelector  OutputSignals=measID
  Constant : Constant  Value=int32(0)
  Constant2 : Constant  Value=int32(1)
  If : If  IfExpression=u1 ~= 0  ShowElse=off
  Selector : Selector  NumberOfDimensions=2  InputPortWidth=3  IndexOptions=Select all,Index vector (port)  Indices=[1 3],1  OutputSizes=1,1
  Switch : Switch  Criteria=u2 ~= 0
  Unit Delay : UnitDelay  InitialCondition=int32(0)  SampleTime=-1
  isValid : Outport
  measID : Outport  Port=2
  nValidMeasCnt : Outport  Port=3
  meas_i : Outport  Port=4
  wires:
  measIdx/1 -> Selector/2
  Selector/1 -> meas_i/1, Bus Selector/1
  measCAN/1 -> Selector/1
  If/1 -> isValid/1
  Switch/1 -> Add/1
  Bus Selector/1 -> measID/1, If/1, Switch/2  "<measID>"
  Constant2/1 -> Switch/1
  Unit Delay/1 -> Add/2
  Constant/1 -> Switch/3
  Add/1 -> nValidMeasCnt/1, Unit Delay/1

== system FusionMODEL_version1/OBJECT_TRACKER_SENSOR_FUSION/SPATIAL_ALLIGNMENT/RADAR_MEASUREMENTS_SPATIAL_ALLIGNMENT/RADAR_MEASUREMENTS_SPATIAL_ALLIGNMENT/COORDINATE_TRANSFORMATION/SET_DATA ==
  measTransformed : Inport
  measID : Inport  Port=2
  RadCANidx : Inport  Port=3
  RadarMeasCAN : Inport  Port=4
  RadarMeasCTSMat : Inport  Port=5
  RadarMeasCTSNoiseMat : Inport  Port=6
  RadarMeasCTSRef : Inport  Port=7
  Assignment1 : Assignment  NumberOfDimensions=2  DiagnosticForDimensions=Warning  IndexOptions=Assign all,Index vector (port)  Indices=1:2,1  OutputSizes=1,1
  Assignment2 : Assignment  NumberOfDimensions=3  DiagnosticForDimensions=Warning  IndexOptions=Assign all,Assign all,Index vector (port)  Indices=1:8,1,1  OutputSizes=1,1,1
  Assignment3 : Assignment  NumberOfDimensions=2  DiagnosticForDimensions=Warning  IndexOptions=Assign all,Index vector (port)  Indices=1:8,1  OutputSizes=1,1
  Bus Selector : BusSelector  OutputSignals=measID,radarID
  Bus Selector1 : BusSelector  OutputSignals=stateCTS,covCTS
  Constant : Constant  Value=single(zeros(2,1))
  Constant1 : Constant  Value=single(zeros(2,2))
  Constant2 : Constant  Value=uint16(zeros(2,1))
  Data Type Conversion : DataTypeConversion  OutDataTypeStr=uint16
  Mux : Mux  Inputs=2
  Reshape : Reshape  OutputDimensionality=Column vector (2-D)
  Switch : Switch  Criteria=u2 ~= 0
  Switch1 : Switch  Criteria=u2 ~= 0
  Switch2 : Switch  Criteria=u2 ~= 0
  Unit Delay : UnitDelay  InitialCondition=single(zeros(2, 200))  SampleTime=-1
  Unit Delay1 : UnitDelay  InitialCondition=single(zeros(2, 2, 200))  SampleTime=-1
  Unit Delay2 : UnitDelay  InitialCondition=uint16(zeros(2, 200))  SampleTime=-1
  RadarCTSMatUpd : Outport
  RadarCTSNoiseCovMatUpd : Outport  Port=2
  RadarCTSRefUpd : Outport  Port=3
  wires:
  RadarMeasCTSMat/1 -> Unit Delay/1
  measID/1 -> Switch/2, Switch2/2, Switch1/2
  Constant/1 -> Switch/3
  Switch/1 -> Assignment1/2
  RadCANidx/1 -> [idx], Assignment1/3
  RadarMeasCAN/1 -> Bus Selector/1
  Unit Delay/1 -> Assignment1/1
  Assignment1/1 -> RadarCTSMatUpd/1
  Bus Selector/1 -> Mux/1  "<measID>"
  Bus Selector/2 -> Data Type Conversion/1  "<radarID>"
  Mux/1 -> Reshape/1
  RadarMeasCTSNoiseMat/1 -> Unit Delay1/1
  Unit Delay1/1 -> Assignment2/1
  Switch1/1 -> Assignment2/2
  measTransformed/1 -> Bus Selector1/1
  Bus Selector1/1 -> Switch/1  "<stateCTS>"
  Constant1/1 -> Switch1/3
  Bus Selector1/2 -> [CTSNoiseCov]  "<covCTS>"
  [CTSNoiseCov] -> Switch1/1
  [idx] -> Assignment2/3
  Switch2/1 -> Assignment3/2
  Constant2/1 -> Switch2/3
  [idx] -> Assignment3/3
  Unit Delay2/1 -> Assignment3/1
  RadarMeasCTSRef/1 -> Unit Delay2/1
  Reshape/1 -> [CTSRef]
  [CTSRef] -> Switch2/1
  Assignment2/1 -> RadarCTSNoiseCovMatUpd/1
  Assignment3/1 -> RadarCTSRefUpd/1
  Data Type Conversion/1 -> Mux/2

== system FusionMODEL_version1/OBJECT_TRACKER_SENSOR_FUSION/SPATIAL_ALLIGNMENT/CAMERA_MEASUREMENTS_SPATIAL_ALLIGNMENT/For Iterator Subsystem/For Iterator Subsystem/CoordinateTransformation1/InfoExtractor ==
  In1 : Inport
  In2 : Inport  Port=2
  Bus Selector : BusSelector  OutputSignals=px,py,vx,vy,NoiseCovarience
  Bus Selector1 : BusSelector  OutputSignals=RotMat2D,TranslationVec
  <px> : Outport
  <py> : Outport  Port=2
  <vx> : Outport  Port=3
  <vy> : Outport  Port=4
  RotMat2D : Outport  Port=5
  TransVec2D : Outport  Port=6
  MeasNoiseCov : Outport  Port=7
  wires:
  Bus Selector/4 -> <vy>/1  "<vy>"
  Bus Selector/2 -> <py>/1  "<py>"
  In1/1 -> Bus Selector/1
  Bus Selector1/1 -> RotMat2D/1  "<RotMat2D>"
  Bus Selector/3 -> <vx>/1  "<vx>"
  Bus Selector1/2 -> TransVec2D/1  "<TranslationVec>"
  Bus Selector/1 -> <px>/1  "<px>"
  In2/1 -> Bus Selector1/1
  Bus Selector/5 -> MeasNoiseCov/1  "<NoiseCovarience>"

== system FusionMODEL_version1/OBJECT_TRACKER_SENSOR_FUSION/SPATIAL_ALLIGNMENT/CAMERA_MEASUREMENTS_SPATIAL_ALLIGNMENT/For Iterator Subsystem/For Iterator Subsystem/CoordinateTransformation1/Meas_Noise_Cov_Transformation ==
  RotMatrix : Inport
  MeasCovarience : Inport  Port=2
  Assignment : Assignment  NumberOfDimensions=2  DiagnosticForDimensions=Warning  IndexOptions=Index vector (dialog),Index vector (dialog)  Indices=[1 2],[1 2]  OutputSizes=1,1
  Assignment1 : Assignment  NumberOfDimensions=2  DiagnosticForDimensions=Warning  IndexOptions=Index vector (dialog),Index vector (dialog)  Indices=[3 4],[3 4]  OutputSizes=1,1
  Matrix Multiply : Product  Inputs=3  Multiplication=Matrix(*)
  Matrix Multiply1 : Product  Inputs=3  Multiplication=Matrix(*)
  Selector : Selector  NumberOfDimensions=2  InputPortWidth=3  IndexOptions=Index vector (dialog),Index vector (dialog)  Indices=[1 2],[1 2]  OutputSizes=1,1
  Selector1 : Selector  NumberOfDimensions=2  InputPortWidth=3  IndexOptions=Index vector (dialog),Index vector (dialog)  Indices=[3 4],[3 4]  OutputSizes=1,1
  Transpose : Math  Operator=transpose  SaturateOnIntegerOverflow=on
  Transpose1 : Math  Operator=transpose  SaturateOnIntegerOverflow=on
  MeasCovTransformed : Outport
  wires:
  Matrix Multiply/1 -> Assignment/2
  [RotationMat] -> Transpose1/1
  Matrix Multiply1/1 -> Assignment1/2
  RotMatrix/1 -> [RotationMat], Matrix Multiply/1
  [NoiseCov] -> Assignment/1
  Transpose1/1 -> Matrix Multiply1/3
  Selector1/1 -> Matrix Multiply1/2
  Assignment/1 -> Assignment1/1
  Selector/1 -> Matrix Multiply/2
  [RotationMat] -> Matrix Multiply1/1, Transpose/1
  Transpose/1 -> Matrix Multiply/3
  MeasCovarience/1 -> Selector1/1, [NoiseCov], Selector/1
  Assignment1/1 -> MeasCovTransformed/1

== system FusionMODEL_version1/OBJECT_TRACKER_SENSOR_FUSION/SPATIAL_ALLIGNMENT/CAMERA_MEASUREMENTS_SPATIAL_ALLIGNMENT/For Iterator Subsystem/For Iterator Subsystem/CoordinateTransformation1/Position_Transformation ==
  Px : Inport
  Py : Inport  Port=2
  RotationMat : Inport  Port=3
  TranslationVector : Inport  Port=4
  Add : Sum
  Matrix Multiply : Product  Multiplication=Matrix(*)
  Mux : Mux  Inputs=2
  Reshape : Reshape  OutputDimensionality=Column vector (2-D)
  Selector : Selector  InputPortWidth=2  IndexOptions=Index vector (dialog)  Indices=1  OutputSizes=1
  Selector1 : Selector  InputPortWidth=2  IndexOptions=Index vector (dialog)  Indices=2  OutputSizes=1
  PosXcts : Outport
  PosYcts : Outport  Port=2
  wires:
  Reshape/1 -> Matrix Multiply/2
  Px/1 -> Mux/1
  Py/1 -> Mux/2
  Mux/1 -> Reshape/1
  RotationMat/1 -> Matrix Multiply/1
  Matrix Multiply/1 -> Add/1
  TranslationVector/1 -> Add/2
  Add/1 -> Selector1/1, Selector/1
  Selector/1 -> PosXcts/1
  Selector1/1 -> PosYcts/1

== system FusionMODEL_version1/OBJECT_TRACKER_SENSOR_FUSION/SPATIAL_ALLIGNMENT/CAMERA_MEASUREMENTS_SPATIAL_ALLIGNMENT/For Iterator Subsystem/For Iterator Subsystem/CoordinateTransformation1/Subsystem ==
  pxCTS : Inport
  pyCTS : Inport  Port=2
  vxCTS : Inport  Port=3
  vyCTS : Inport  Port=4
  covCTS : Inport  Port=5
  Bus Creator : BusCreator  Inputs=2
  Mux : Mux  Inputs=2
  Reshape : Reshape  OutputDimensionality=Column vector (2-D)
  Selector : Selector  NumberOfDimensions=2  InputPortWidth=3  IndexOptions=Index vector (dialog),Index vector (dialog)  Indices=1:2,1:2  OutputSizes=1,1
  Terminator : Terminator
  Terminator1 : Terminator
  measUpd : Outport
  wires:
  covCTS/1 -> Selector/1
  Bus Creator/1 -> measUpd/1
  pyCTS/1 -> Mux/2
  pxCTS/1 -> Mux/1
  Mux/1 -> Reshape/1
  Reshape/1 -> Bus Creator/1  "stateCTS"
  Selector/1 -> Bus Creator/2  "covCTS"
  vxCTS/1 -> Terminator/1
  vyCTS/1 -> Terminator1/1

== system FusionMODEL_version1/OBJECT_TRACKER_SENSOR_FUSION/SPATIAL_ALLIGNMENT/CAMERA_MEASUREMENTS_SPATIAL_ALLIGNMENT/For Iterator Subsystem/For Iterator Subsystem/CoordinateTransformation1/Velocity_Transformation ==
  Vx : Inport
  Vy : Inport  Port=2
  RotMatrix2D : Inport  Port=3
  Matrix Multiply : Product  Multiplication=Matrix(*)
  Mux : Mux  Inputs=2
  Reshape : Reshape  OutputDimensionality=Column vector (2-D)
  Selector : Selector  InputPortWidth=2  IndexOptions=Index vector (dialog)  Indices=1  OutputSizes=1
  Selector1 : Selector  InputPortWidth=2  IndexOptions=Index vector (dialog)  Indices=2  OutputSizes=1
  VelXcts : Outport
  VelYcts : Outport  Port=2
  wires:
  Vy/1 -> Mux/2
  RotMatrix2D/1 -> Matrix Multiply/1
  Vx/1 -> Mux/1
  Mux/1 -> Reshape/1
  Reshape/1 -> Matrix Multiply/2
  Matrix Multiply/1 -> Selector1/1, Selector/1
  Selector/1 -> VelXcts/1
  Selector1/1 -> VelYcts/1

== system FusionMODEL_version1/OBJECT_TRACKER_SENSOR_FUSION/SPATIAL_ALLIGNMENT/RADAR_MEASUREMENTS_SPATIAL_ALLIGNMENT/RADAR_MEASUREMENTS_SPATIAL_ALLIGNMENT/COORDINATE_TRANSFORMATION/COORDINATE_TRANSFORMATION/GET_DATA ==
  In1 : Inport
  In2 : Inport  Port=2
  Bus Selector : BusSelector  OutputSignals=px,py,vx,vy,NoiseCovarience
  Bus Selector1 : BusSelector  OutputSignals=RotMat2D,TranslationVec
  <px> : Outport
  <py> : Outport  Port=2
  <vx> : Outport  Port=3
  <vy> : Outport  Port=4
  RotMat2D : Outport  Port=5
  TransVec2D : Outport  Port=6
  MeasNoiseCov : Outport  Port=7
  wires:
  Bus Selector/4 -> <vy>/1  "<vy>"
  Bus Selector/2 -> <py>/1  "<py>"
  In1/1 -> Bus Selector/1
  Bus Selector1/1 -> RotMat2D/1  "<RotMat2D>"
  Bus Selector/3 -> <vx>/1  "<vx>"
  Bus Selector1/2 -> TransVec2D/1  "<TranslationVec>"
  Bus Selector/1 -> <px>/1  "<px>"
  In2/1 -> Bus Selector1/1
  Bus Selector/5 -> MeasNoiseCov/1  "<NoiseCovarience>"

== system FusionMODEL_version1/OBJECT_TRACKER_SENSOR_FUSION/SPATIAL_ALLIGNMENT/RADAR_MEASUREMENTS_SPATIAL_ALLIGNMENT/RADAR_MEASUREMENTS_SPATIAL_ALLIGNMENT/COORDINATE_TRANSFORMATION/COORDINATE_TRANSFORMATION/MEAS_NOISE_COV_TRANSFORMATION ==
  RotMatrix : Inport
  MeasCovarience : Inport  Port=2
  Assignment : Assignment  NumberOfDimensions=2  DiagnosticForDimensions=Warning  IndexOptions=Index vector (dialog),Index vector (dialog)  Indices=[1 2],[1 2]  OutputSizes=1,1
  Assignment1 : Assignment  NumberOfDimensions=2  DiagnosticForDimensions=Warning  IndexOptions=Index vector (dialog),Index vector (dialog)  Indices=[3 4],[3 4]  OutputSizes=1,1
  Matrix Multiply : Product  Inputs=3  Multiplication=Matrix(*)
  Matrix Multiply1 : Product  Inputs=3  Multiplication=Matrix(*)
  Selector : Selector  NumberOfDimensions=2  InputPortWidth=3  IndexOptions=Index vector (dialog),Index vector (dialog)  Indices=[1 2],[1 2]  OutputSizes=1,1
  Selector1 : Selector  NumberOfDimensions=2  InputPortWidth=3  IndexOptions=Index vector (dialog),Index vector (dialog)  Indices=[3 4],[3 4]  OutputSizes=1,1
  Transpose : Math  Operator=transpose  SaturateOnIntegerOverflow=on
  Transpose1 : Math  Operator=transpose  SaturateOnIntegerOverflow=on
  MeasCovTransformed : Outport
  wires:
  Matrix Multiply/1 -> Assignment/2
  [RotationMat] -> Transpose1/1
  Matrix Multiply1/1 -> Assignment1/2
  RotMatrix/1 -> [RotationMat], Matrix Multiply/1
  [NoiseCov] -> Assignment/1
  Transpose1/1 -> Matrix Multiply1/3
  Selector1/1 -> Matrix Multiply1/2
  Assignment/1 -> Assignment1/1
  Selector/1 -> Matrix Multiply/2
  [RotationMat] -> Matrix Multiply1/1, Transpose/1
  Transpose/1 -> Matrix Multiply/3
  MeasCovarience/1 -> Selector1/1, [NoiseCov], Selector/1
  Assignment1/1 -> MeasCovTransformed/1

== system FusionMODEL_version1/OBJECT_TRACKER_SENSOR_FUSION/SPATIAL_ALLIGNMENT/RADAR_MEASUREMENTS_SPATIAL_ALLIGNMENT/RADAR_MEASUREMENTS_SPATIAL_ALLIGNMENT/COORDINATE_TRANSFORMATION/COORDINATE_TRANSFORMATION/POSITION_TRANSFORMATION ==
  Px : Inport
  Py : Inport  Port=2
  RotationMat : Inport  Port=3
  TranslationVector : Inport  Port=4
  Add : Sum
  Matrix Multiply : Product  Multiplication=Matrix(*)
  Mux : Mux  Inputs=2
  Reshape : Reshape  OutputDimensionality=Column vector (2-D)
  Selector : Selector  InputPortWidth=2  IndexOptions=Index vector (dialog)  Indices=1  OutputSizes=1
  Selector1 : Selector  InputPortWidth=2  IndexOptions=Index vector (dialog)  Indices=2  OutputSizes=1
  PosXcts : Outport
  PosYcts : Outport  Port=2
  wires:
  Reshape/1 -> Matrix Multiply/2
  Px/1 -> Mux/1
  Py/1 -> Mux/2
  Mux/1 -> Reshape/1
  RotationMat/1 -> Matrix Multiply/1
  Matrix Multiply/1 -> Add/1
  TranslationVector/1 -> Add/2
  Add/1 -> Selector1/1, Selector/1
  Selector/1 -> PosXcts/1
  Selector1/1 -> PosYcts/1

== system FusionMODEL_version1/OBJECT_TRACKER_SENSOR_FUSION/SPATIAL_ALLIGNMENT/RADAR_MEASUREMENTS_SPATIAL_ALLIGNMENT/RADAR_MEASUREMENTS_SPATIAL_ALLIGNMENT/COORDINATE_TRANSFORMATION/COORDINATE_TRANSFORMATION/SET_DATA ==
  pxCTS : Inport
  pyCTS : Inport  Port=2
  vxCTS : Inport  Port=3
  vyCTS : Inport  Port=4
  covCTS : Inport  Port=5
  Bus Creator : BusCreator  Inputs=2
  Mux : Mux  Inputs=2
  Reshape : Reshape  OutputDimensionality=Column vector (2-D)
  Selector : Selector  NumberOfDimensions=2  InputPortWidth=3  IndexOptions=Index vector (dialog),Index vector (dialog)  Indices=1:2,1:2  OutputSizes=1,1
  Terminator : Terminator
  Terminator1 : Terminator
  measUpd : Outport
  wires:
  covCTS/1 -> Selector/1
  Bus Creator/1 -> measUpd/1
  pyCTS/1 -> Mux/2
  pxCTS/1 -> Mux/1
  Mux/1 -> Reshape/1
  Reshape/1 -> Bus Creator/1  "stateCTS"
  Selector/1 -> Bus Creator/2  "covCTS"
  vxCTS/1 -> Terminator/1
  vyCTS/1 -> Terminator1/1

== system FusionMODEL_version1/OBJECT_TRACKER_SENSOR_FUSION/SPATIAL_ALLIGNMENT/RADAR_MEASUREMENTS_SPATIAL_ALLIGNMENT/RADAR_MEASUREMENTS_SPATIAL_ALLIGNMENT/COORDINATE_TRANSFORMATION/COORDINATE_TRANSFORMATION/VELOCITY_TRANSFORMATION ==
  Vx : Inport
  Vy : Inport  Port=2
  RotMatrix2D : Inport  Port=3
  Matrix Multiply : Product  Multiplication=Matrix(*)
  Mux : Mux  Inputs=2
  Reshape : Reshape  OutputDimensionality=Column vector (2-D)
  Selector : Selector  InputPortWidth=2  IndexOptions=Index vector (dialog)  Indices=1  OutputSizes=1
  Selector1 : Selector  InputPortWidth=2  IndexOptions=Index vector (dialog)  Indices=2  OutputSizes=1
  VelXcts : Outport
  VelYcts : Outport  Port=2
  wires:
  Vy/1 -> Mux/2
  RotMatrix2D/1 -> Matrix Multiply/1
  Vx/1 -> Mux/1
  Mux/1 -> Reshape/1
  Reshape/1 -> Matrix Multiply/2
  Matrix Multiply/1 -> Selector1/1, Selector/1
  Selector/1 -> VelXcts/1
  Selector1/1 -> VelYcts/1

== matlab function FusionMODEL_version1/OBJECT_TRACKER_SENSOR_FUSION/SPATIAL_ALLIGNMENT/RADAR_MEASUREMENTS_SPATIAL_ALLIGNMENT/SET_MEASUREMENTS/FindNonZeroIndex ==
  data: idx_in input; idx output
function idx = fcn(idx_in)
    idx = int32(zeros(1,length(idx_in)));
    validIdxCnt = length(idx);
    if validIdxCnt ~= 0 
       MeasIdx = find(idx_in ~= uint16(0));
       idx(1,1:validIdxCnt) = MeasIdx;
    end
end
